simulink model "test_kinematic_transform_sim"  (R2021b)
settings: Solver=VariableStepAuto  StartTime=0.0  StopTime=10.0  RelTol=1e-3
libraries: my_math_ops x2, kinematic_transform x1
settings Model: Creator=Davide  LastModifiedBy=Davide

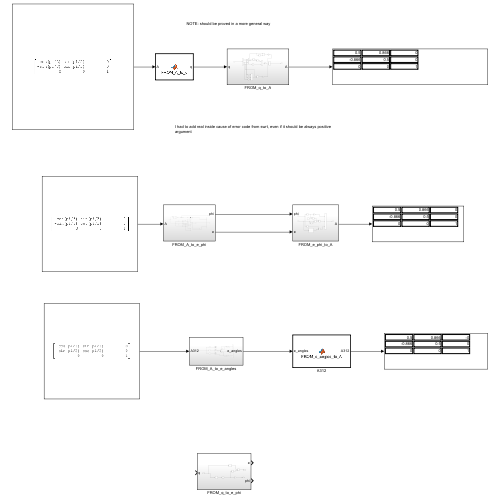
[thumbnail: Simulink's stored preview of the top-level diagram]
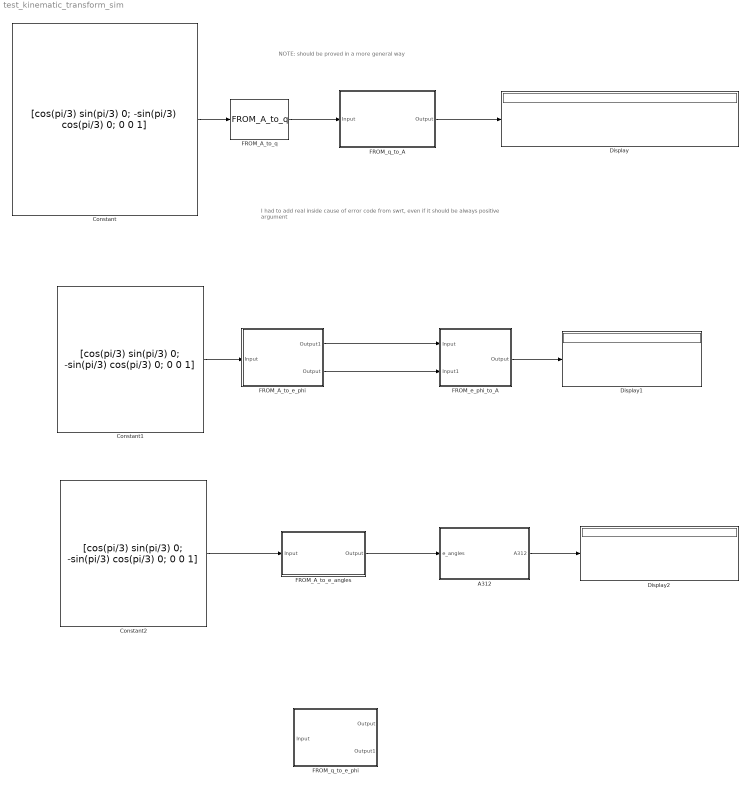
== system test_kinematic_transform_sim ==
  note: I had to add real inside cause of error code from swrt, even if it should be always positive argument
  note: NOTE: should be proved in a more general way
  A312 : MATLAB Function  TreatAsAtomicUnit=on
  Constant : Constant  Value=[cos(pi/3) sin(pi/3) 0; -sin(pi/3) cos(pi/3) 0; 0 0 1]
  Constant1 : Constant  Value=[cos(pi/3) sin(pi/3) 0; -sin(pi/3) cos(pi/3) 0; 0 0 1]
  Constant2 : Constant  Value=[cos(pi/3) sin(pi/3) 0; -sin(pi/3) cos(pi/3) 0; 0 0 1]
  Display : Display
  Display1 : Display
  Display2 : Display
  FROM_A_to_e_angles : Subsystem
  FROM_A_to_e_phi : Subsystem
  FROM_A_to_q : kinematic_transform/FROM_A_to_q  SystemSampleTime=-1  VariantActivationTime=update diagram  Latency=0  AutoFrameSizeCalculation=off
      settings: SourceProductName=Kinematic Transformation
  FROM_e_phi_to_A : Subsystem
  FROM_q_to_A : Subsystem
  FROM_q_to_e_phi : Subsystem
  wires:
  FROM_A_to_q/1 -> FROM_q_to_A/1(Input)
  Constant/1 -> FROM_A_to_q/1
  FROM_q_to_A/1(Output) -> Display/1
  Constant1/1 -> FROM_A_to_e_phi/1(Input)
  FROM_e_phi_to_A/1(Output) -> Display1/1
  FROM_A_to_e_phi/1(Output1) -> FROM_e_phi_to_A/1(Input)
  FROM_A_to_e_phi/2(Output) -> FROM_e_phi_to_A/2(Input1)
  FROM_A_to_e_angles/1(Output) -> A312/1(e_angles)
  Constant2/1 -> FROM_A_to_e_angles/1(Input)
  A312/1(A312) -> Display2/1

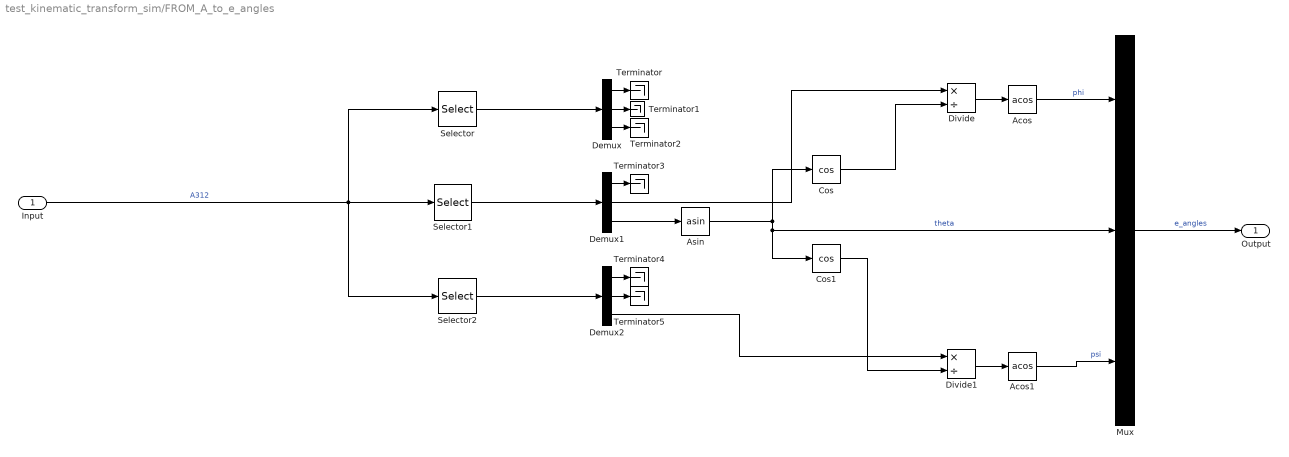
== system test_kinematic_transform_sim/FROM_A_to_e_angles ==
  Input : Inport
  Acos : Trigonometry  Operator=acos
  Acos1 : Trigonometry  Operator=acos
  Asin : Trigonometry  Operator=asin
  Cos : Trigonometry  Operator=cos
  Cos1 : Trigonometry  Operator=cos
  Demux : Demux  Outputs=3
  Demux1 : Demux  Outputs=3
  Demux2 : Demux  Outputs=3
  Divide : Product  Inputs=*/
  Divide1 : Product  Inputs=*/
  Mux : Mux  Inputs=3
  Selector : Selector  NumberOfDimensions=2  InputPortWidth=3  IndexOptions=Index vector (dialog),Select all  Indices=1,1  OutputSizes=1,1
  Selector1 : Selector  NumberOfDimensions=2  InputPortWidth=3  IndexOptions=Index vector (dialog),Select all  Indices=2,1  OutputSizes=1,1
  Selector2 : Selector  NumberOfDimensions=2  InputPortWidth=3  IndexOptions=Index vector (dialog),Select all  Indices=3,1  OutputSizes=1,1
  Terminator{,1..5} (6 alike) : Terminator
  Output : Outport
  wires:
  Mux/1 -> Output/1  "e_angles"
  Asin/1 -> Cos1/1, Mux/2, Cos/1  "theta"
  Divide/1 -> Acos/1
  Selector/1 -> Demux/1
  Demux2/3 -> Divide1/1
  Selector2/1 -> Demux2/1
  Input/1 -> Selector2/1, Selector/1, Selector1/1  "A312"
  Acos1/1 -> Mux/3  "psi"
  Cos/1 -> Divide/2
  Selector1/1 -> Demux1/1
  Demux1/1 -> Terminator3/1
  Demux1/2 -> Divide/1
  Divide1/1 -> Acos1/1
  Cos1/1 -> Divide1/2
  Demux1/3 -> Asin/1
  Acos/1 -> Mux/1  "phi"
  Demux/2 -> Terminator1/1
  Demux/3 -> Terminator2/1
  Demux2/2 -> Terminator5/1
  Demux2/1 -> Terminator4/1
  Demux/1 -> Terminator/1

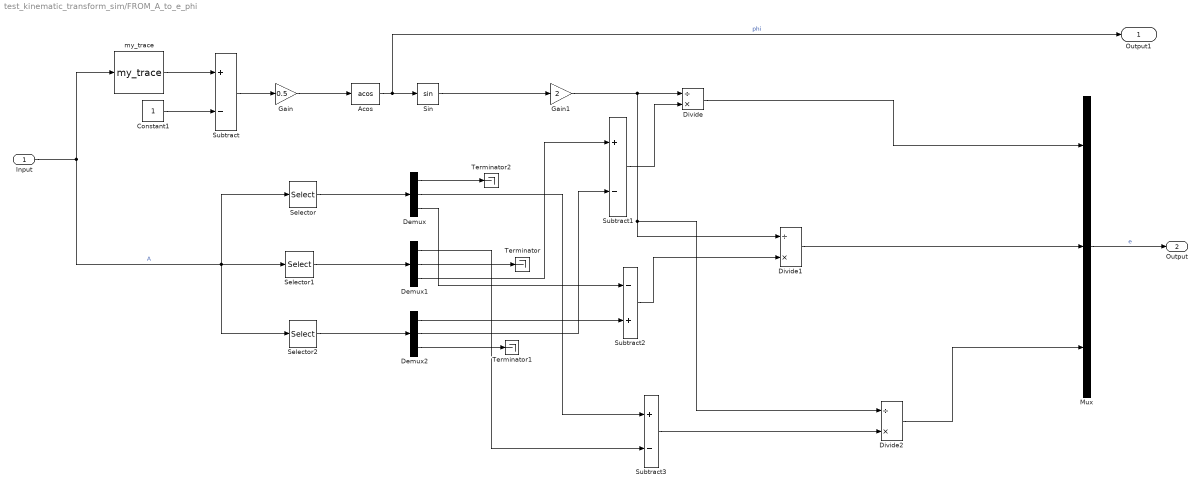
== system test_kinematic_transform_sim/FROM_A_to_e_phi ==
  Input : Inport
  Acos : Trigonometry  Operator=acos
  Constant1 : Constant
  Demux : Demux  Outputs=3
  Demux1 : Demux  Outputs=3
  Demux2 : Demux  Outputs=3
  Divide : Product  Inputs=/*
  Divide1 : Product  Inputs=/*
  Divide2 : Product  Inputs=/*
  Gain : Gain  Gain=0.5
  Gain1 : Gain  Gain=2
  Mux : Mux  Inputs=3
  Selector : Selector  NumberOfDimensions=2  InputPortWidth=3  IndexOptions=Index vector (dialog),Select all  Indices=1,1  OutputSizes=1,1
  Selector1 : Selector  NumberOfDimensions=2  InputPortWidth=3  IndexOptions=Index vector (dialog),Select all  Indices=2,1  OutputSizes=1,1
  Selector2 : Selector  NumberOfDimensions=2  InputPortWidth=3  IndexOptions=Index vector (dialog),Select all  Indices=3,1  OutputSizes=1,1
  Sin : Trigonometry
  Subtract : Sum  Inputs=+-
  Subtract1 : Sum  Inputs=+-
  Subtract2 : Sum  Inputs=-+
  Subtract3 : Sum  Inputs=+-
  Terminator : Terminator
  Terminator1 : Terminator
  Terminator2 : Terminator
  my_trace : my_math_ops/my_trace  SystemSampleTime=-1  VariantActivationTime=update diagram  Latency=0  AutoFrameSizeCalculation=off
      settings: SourceProductName=My Mathematics Operations
  Output1 : Outport
  Output : Outport  Port=2
  wires:
  Demux1/3 -> Subtract1/1
  Demux/1 -> Terminator2/1
  Divide1/1 -> Mux/2
  Demux2/2 -> Subtract1/2
  Demux/2 -> Subtract3/1
  Demux1/1 -> Subtract3/2
  Demux2/1 -> Subtract2/2
  Sin/1 -> Gain1/1
  Subtract3/1 -> Divide2/2
  Input/1 -> Selector2/1, Selector/1, Selector1/1, my_trace/1  "A"
  Constant1/1 -> Subtract/2
  Acos/1 -> Output1/1, Sin/1  "phi"
  Gain1/1 -> Divide2/1, Divide1/1, Divide/1
  Selector/1 -> Demux/1
  Demux1/2 -> Terminator/1
  Subtract2/1 -> Divide1/2
  my_trace/1 -> Subtract/1
  Divide2/1 -> Mux/3
  Subtract/1 -> Gain/1
  Mux/1 -> Output/1  "e"
  Divide/1 -> Mux/1
  Gain/1 -> Acos/1
  Selector1/1 -> Demux1/1
  Demux/3 -> Subtract2/1
  Selector2/1 -> Demux2/1
  Subtract1/1 -> Divide/2
  Demux2/3 -> Terminator1/1

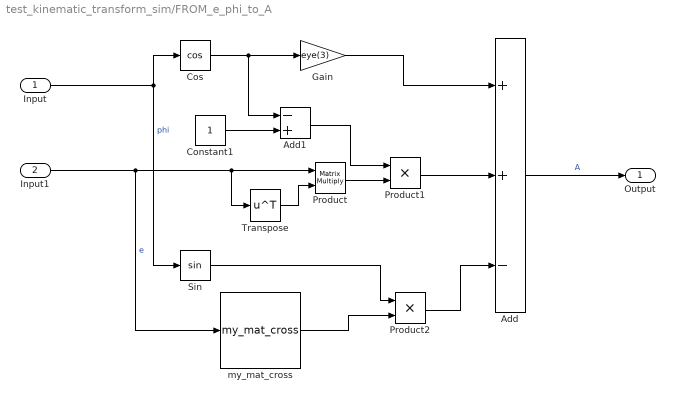
== system test_kinematic_transform_sim/FROM_e_phi_to_A ==
  Input : Inport
  Input1 : Inport  Port=2
  Add : Sum  Inputs=++-
  Add1 : Sum  Inputs=-+
  Constant1 : Constant
  Cos : Trigonometry  Operator=cos
  Gain : Gain  Gain=eye(3)
  Product : Product  Multiplication=Matrix(*)
  Product1 : Product
  Product2 : Product
  Sin : Trigonometry
  Transpose : Math  Operator=transpose  SaturateOnIntegerOverflow=on
  my_mat_cross : my_math_ops/my_mat_cross  SystemSampleTime=-1  VariantActivationTime=update diagram  Latency=0  AutoFrameSizeCalculation=off
      settings: SourceProductName=My Mathematics Operations
  Output : Outport
  wires:
  Sin/1 -> Product2/1
  Add/1 -> Output/1  "A"
  my_mat_cross/1 -> Product2/2
  Gain/1 -> Add/1
  Input1/1 -> my_mat_cross/1, Transpose/1, Product/1  "e"
  Product/1 -> Product1/2
  Constant1/1 -> Add1/2
  Product2/1 -> Add/3
  Cos/1 -> Add1/1, Gain/1
  Add1/1 -> Product1/1
  Input/1 -> Sin/1, Cos/1  "phi"
  Transpose/1 -> Product/2
  Product1/1 -> Add/2

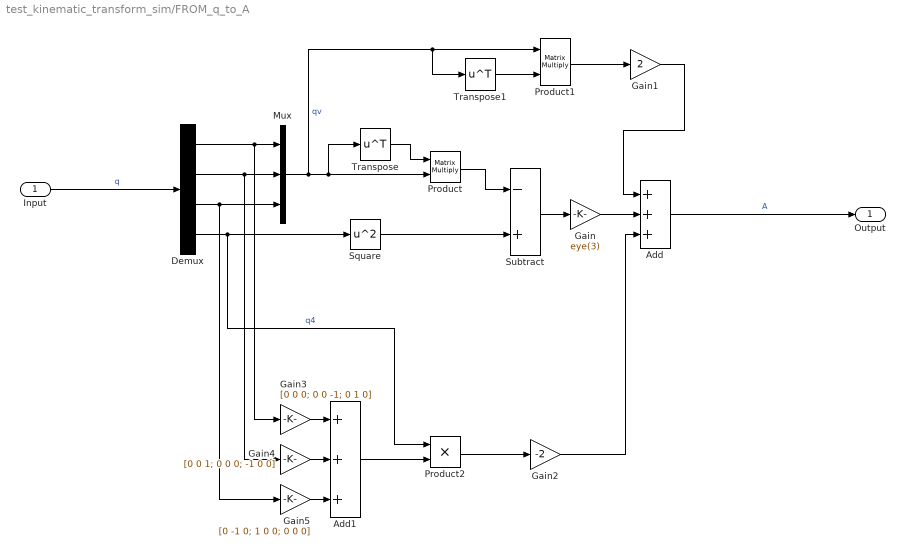
== system test_kinematic_transform_sim/FROM_q_to_A ==
  Input : Inport
  Add : Sum  Inputs=+++
  Add1 : Sum  Inputs=+++
  Demux : Demux
  Gain : Gain  Gain=eye(3)
  Gain1 : Gain  Gain=2
  Gain2 : Gain  Gain=-2
  Gain3 : Gain  Gain=[0 0 0; 0 0 -1; 0 1 0]
  Gain4 : Gain  Gain=[0 0 1; 0 0 0; -1 0 0]
  Gain5 : Gain  Gain=[0 -1 0; 1 0 0; 0 0 0]
  Mux : Mux  Inputs=3
  Product : Product  Multiplication=Matrix(*)
  Product1 : Product  Multiplication=Matrix(*)
  Product2 : Product
  Square : Math  Operator=square  SaturateOnIntegerOverflow=on
  Subtract : Sum  Inputs=-+
  Transpose : Math  Operator=transpose  SaturateOnIntegerOverflow=on
  Transpose1 : Math  Operator=transpose  SaturateOnIntegerOverflow=on
  Output : Outport
  wires:
  Mux/1 -> Transpose1/1, Product1/1, Product/2, Transpose/1  "qv"
  Demux/4 -> Product2/1, Square/1  "q4"
  Square/1 -> Subtract/2
  Add/1 -> Output/1  "A"
  Demux/1 -> Gain3/1, Mux/1
  Demux/2 -> Gain4/1, Mux/2
  Product/1 -> Subtract/1
  Gain4/1 -> Add1/2
  Transpose/1 -> Product/1
  Product1/1 -> Gain1/1
  Transpose1/1 -> Product1/2
  Demux/3 -> Gain5/1, Mux/3
  Gain/1 -> Add/2
  Product2/1 -> Gain2/1
  Gain1/1 -> Add/1
  Subtract/1 -> Gain/1
  Input/1 -> Demux/1  "q"
  Gain2/1 -> Add/3
  Gain5/1 -> Add1/3
  Gain3/1 -> Add1/1
  Add1/1 -> Product2/2

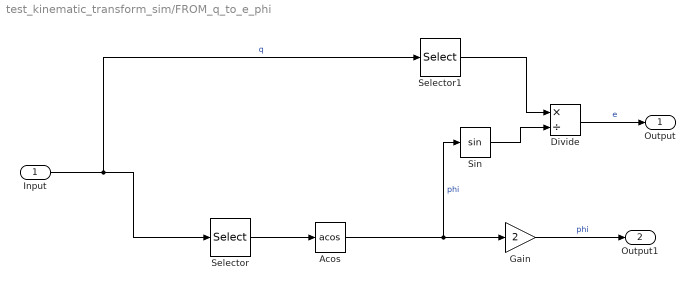
== system test_kinematic_transform_sim/FROM_q_to_e_phi ==
  Input : Inport
  Acos : Trigonometry  Operator=acos
  Divide : Product  Inputs=*/
  Gain : Gain  Gain=2
  Selector : Selector  InputPortWidth=4  IndexOptions=Index vector (dialog)  Indices=4  OutputSizes=1
  Selector1 : Selector  InputPortWidth=4  IndexOptions=Index vector (dialog)  Indices=[1 2 3]  OutputSizes=1
  Sin : Trigonometry
  Output : Outport
  Output1 : Outport  Port=2
  wires:
  Sin/1 -> Divide/2
  Selector/1 -> Acos/1
  Selector1/1 -> Divide/1
  Acos/1 -> Gain/1, Sin/1  "phi"
  Input/1 -> Selector1/1, Selector/1  "q"
  Divide/1 -> Output/1  "e"
  Gain/1 -> Output1/1  "phi"

== matlab function test_kinematic_transform_sim/A312 ==
  data: e_angles input; A312 output
function A312 = FROM_e_angles_to_A(e_angles)
phi = e_angles(1);
theta = e_angles(2);
psi = e_angles(3);
A312 = [cos(psi)*cos(phi)-sin(psi)*sin(phi)*sin(theta), cos(psi)*sin(phi) + sin(psi)*cos(phi)*sin(theta), -sin(psi)*cos(theta);
     -sin(phi)*cos(theta), cos(phi)*cos(theta), sin(theta);
     sin(psi)*cos(phi)+cos(psi)*sin(phi)*sin(theta), sin(psi)*sin(phi)-cos(psi)*cos(phi)*sin(theta), cos(theta)*cos(psi)];
end
